simulink model "EDS1"  (R2023a)
settings: Solver=VariableStepAuto  StartTime=0.0  StopTime=600  RelTol=1e-3
undefined symbols (not defined in the file): Ion, Lithium
libraries: spsBatteryLib x2, spsDCMachineLib x2, spspowerguiLib x1
settings Model: PacingRate=0.011000  Creator=mluser  LastModifiedBy=Channaveera Gouda

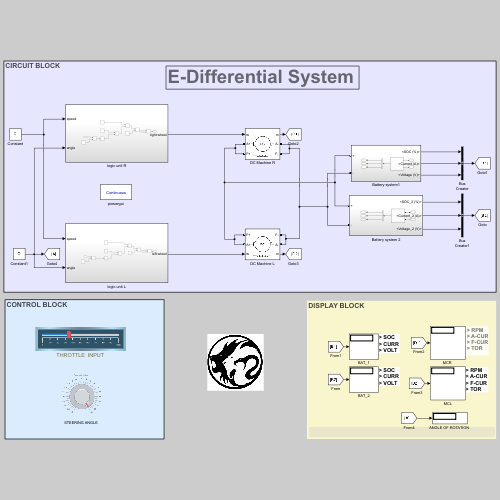
[thumbnail: Simulink's stored preview of the top-level diagram]
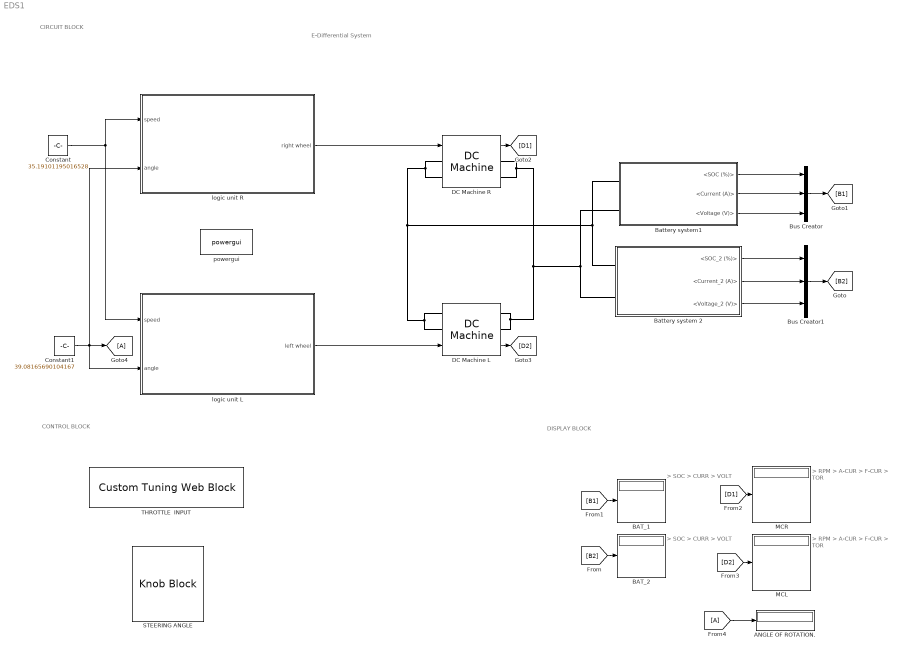
== system EDS1 ==
  note: CONTROL BLOCK
  note: DISPLAY BLOCK
  note: CIRCUIT BLOCK
  note: > RPM
      | > A-CUR
      | > F-CUR
      | > TOR
  note: > RPM
      | > A-CUR
      | > F-CUR
      | > TOR
  note: E-Differential System
  note: > SOC
      | > CURR
      | > VOLT
  note: > SOC
      | > CURR
      | > VOLT
  ANGLE OF ROTATION. : Display
  BAT_1 : Display
  BAT_2 : Display
  Battery system 2 : Subsystem
  Battery system1 : Subsystem
  Bus Creator : BusCreator  Inputs=3
  Bus Creator1 : BusCreator  Inputs=3
  Constant : Constant  Value=35.19101195016528
  Constant1 : Constant  Value=39.08165690104167
  DC Machine L : spsDCMachineLib/DC Machine  PresetModel=01: 5HP 240V 1750RPM Field:300V  MechanicalLoad=Speed w  FieldType=Wound  ShowDetailedParameters=on  MeasurementBus=off  RLa=[2.581 0.028]  RLf=[281.2 156]  Laf=0.9483  MachineConstant=Torque constant (N.m/A)  Ke=1.8  Kt=1.8  J=0.02215  Bm=0.002953  Tf=0.5161  w0=1  Ifinit=0  TsPowergui=0  TsBlock=-1
  DC Machine R : spsDCMachineLib/DC Machine  PresetModel=01: 5HP 240V 1750RPM Field:300V  MechanicalLoad=Speed w  FieldType=Wound  ShowDetailedParameters=on  MeasurementBus=off  RLa=[2.581 0.028]  RLf=[281.2 156]  Laf=0.9483  MachineConstant=Torque constant (N.m/A)  Ke=1.8  Kt=1.8  J=0.02215  Bm=0.002953  Tf=0.5161  w0=1  Ifinit=0  TsPowergui=0  TsBlock=-1
  From4 : From
  Goto4 : Goto
  MCL : Display
  "MCR " : Display
  STEERING ANGLE : KnobBlock  ScaleMin=-40  ScaleMax=40
  THROTTLE  INPUT : CustomTuningWebBlock  LabelPosition=Hide  ShowInitialText=on  Configuration="{\"components\":[{\"name\":\"LinearScaleComponent\",\"settings\":{\"bounds\":{\"max\":100,\"min\":0,\"tickInterval\":\"auto\"},\"internalTickHeightScaleFactor\":0.5,\"labelColor\":[255,255,200],\"labelFont\":{\"font\":\"Arial\",\"fontSize\":12},\"labelOffset\":0.05,\"labelTransparency\":1,\"needleImage\":{\"size\":[596,842],\"src\":\"data:image\\/svg+xml;base64,PD94bWwgdmVyc2lvbj0iMS4wIiBlbmNvZGluZz0idXRmLTgiPz4NCjwhLS0gR2VuZXJhdG9yOiBBZG9iZSBJbGx1c3RyYXRvciAyNS4wLjAsIFNWRyBFeHBvcnQgUGx1Zy1JbiAuIFNWRyBWZXJzaW9uOiA2LjAwIEJ1aWxkIDApICAtLT4NCjxzdmcgdmVyc2lvbj0iMS4xIg0KCSBpZD0ic3ZnOCIgeG1sbnM6Y2M9Imh0dHA6Ly9jcmVhdGl2ZWNvbW1vbnMub3JnL25zIyIgeG1sbnM6ZGM9Imh0dHA6Ly9wdXJsLm9yZy9kYy9lbGVtZW50cy8xLjEvIiB4bWxuczppbmtzY2FwZT0iaHR0cDovL3d3dy5pbmtzY2FwZS5vcmcvbmFtZXNw ...(+2420 chars)\",\"srcOrientation\":\"Right\"},\"needleOffset\":[-0.8044596912521441,-0.0642123287671233],\"needleSize\":{\"height\":0.4337797619047619,\"width\":0.07668067226890757},\"position\":[0.2829861111111111,0.04398634453781513,0.9196428571428571,0.6088789682539683],\"referencePoint\":\"auto\",\"scaleColors\":[],\"scaleColorsSize\":0.2,\"scaleDirection\":\"LR\",\"showLabels\":1,\"showMinorTicks\":0,\"showSpanLine\":1,\"showTicks\":1,\"tickColor\":[252,252,197],\"tickTransparency\":1,\"valueBarColor\":[0,114,189],\"valueBarOffset\":-0.27,\"valueBarSize\":0.1,\"valueBarTransparency\":1}},{\"name\":\"BackgroundImageComponent\",\"settings\":{\"image\":{\"size\":[380,101],\"src\":\"data:image\\/svg+xml;base64,PHN2ZyB4bWxucz0iaHR0cDovL3d3dy53My5vcmcvMjAwMC9zdmciIHhtbG5zOnhsaW5rPSJodHRwOi8vd3d3LnczLm9yZy8xOTk5L3hsaW5rIiB2aWV3Qm94PSIwIDAgMzgwIDEwMSI+PGRlZnM+PHN0eWxlPi5jbHMtMXtmaWxsOiMwMDJiNDI7fS5jbHMtMntmaWxsOiM0MjcwODI7fS5jbHMtM3tmaWxsOnVybCgjcmFkaWFsLWdyYWRpZW50KTt9LmNscy00e2ZpbGw6I2M4YzhjODtzdHJva2U6IzAwMDt9PC9zdHlsZT48cmFkaWFsR3JhZGllbnQgaWQ9InJhZGlhbC1ncmFkaWVudCIgY3g9IjE5MCIgY3k9IjUwLjUiIHI9IjI2OS4yMSIgZ3JhZGllbnRVbml0cz0idXNlclNwYWNlT25Vc2UiPjxzdG9wIG9mZnNldD0iMC4wMSIgc3RvcC1jb2xvcj0iIzNlNGY1OCIvPjxzdG9wIG9mZnNldD0iMC4wNiIgc3RvcC1jb2xvcj0iIzQ0NTc2MSIvPjxzdG9wIG9mZnNldD0iMC4xNSIgc3RvcC1jb2xvcj0iIzU1NmE3NiIvPjxzdG9wIG9mZnNldD0iMC4yNSIgc3RvcC1jb2xvcj0iIzZkODg5NSIvPjxzdG9wIG9mZnNldD0iMC4zOCIgc3RvcC1jb2xvcj0iIzhmYjJjMyIvPjxzdG9wIG9mZnNldD0iMC41MiIgc3RvcC1jb2xvcj0iI2I2ZTRmYSIvPjxzdG9wIG9mZnNldD0iMSIgc3RvcC1jb2xvcj0iIzE1NDY1NyIvPjwvcmFkaWFsR3JhZGllbnQ+PC9kZWZzPjxnIGlkPSJmcmFtZSI+PGcgaWQ9IkxheWVyXzIiIGRhdGEtbmFtZT0iTGF5ZXIgMiI+PGcgaWQ9IkxheWVyXzEtMiIgZGF0YS1uYW1lPSJMYXllciAxLTIiPjxyZWN0IGlkPSJyZWN0MTAzNiIgY2xhc3M9ImNscy0xIiB4PSIxMSIgeT0iMTEiIHdpZHRoPSIzNTgiIGhlaWdodD0iNzkiLz48cGF0aCBpZD0icGF0aDEwMzgiIGNsYXNzPSJjbHMtMiIgZD0iTTgsOFY5M0gzNzJWOFpNMzY5LDkwSDExVjExSDM2OVoiLz48cGF0aCBpZD0icGF0aDEwNDAiIGNsYXNzPSJjbHMtMyIgZD0iTTAsMFYxMDFIMzgwVjBaTTM3Miw5M0g4VjhIMzcyWiIvPjwvZz48L2c+PC9nPjxnIGlkPSJ0cmFjayI+PHBhdGggaWQ9InJlY3QxNjExIiBjbGFzcz0iY2xzLTQiIGQ9Ik0zMy4zNywyNi41OUgzNDYuNjNjNCwwLDcuMjUsMi42LDcuMjUsNS44MWgwYzAsMy4yMS0zLjI1LDUuODItNy4yNSw1LjgySDMzLjM3Yy00LDAtNy4yNS0yLjYxLTcuMjUtNS44MmgwQzI2LjEyLDI5LjE5LDI5LjM3LDI2LjU5LDMzLjM3LDI2LjU5WiIvPjwvZz48L3N2Zz4=\",\"srcOrientation\":\"horizontal\"},\"position\":[0,0,1,1],\"scaleMode\":\"0\"}},{\"name\":\"ForegroundImageComponent\",\"settings\":{\"image\":{\"size\":[0,0],\"src\":\"default\",\"srcOrientation\":[]},\"isForeground\":1,\"position\":[0,0,1,1],\"scaleMode\":\"0\"}}],\"settings\":{\"BindingType\":\"param\",\"aspectRatio\":3.7777777777777777,\"backgroundColor\":[0,0,0,\"1\"],\"backgroundOffset\":0,\"backgroundOpacity\":1,\"fixedAspectRatio\":\"on\",\"foregroundColor\":[252,252,196],\"orientation\":\"horizontal\",\"showBackgroundColor\":false,\"value\":0,\"version\":\"R2023a\"},\"type\":\"LinearGauge\"}"
  logic unit L : Subsystem
  logic unit R : Subsystem
  powergui : spspowerguiLib/powergui  Priority=1  SimulationMode=Continuous  SampleTime=50e-6  frequency=60  Iterations=50  frequencyindice=0  Pbase=100e6  ErrMax=1e-4  UnitsV=kV  UnitsW=MW  buscounter=0  FunctionMessages=off  echomessages=off  EnableUseOfTLC=off  CurrentSourceSwitches=off  DisableSnubberDevices=off  DisableRonSwitches=off  DisableVfSwitches=off  DisplayEquations=off  AutomaticDiscreteSolvers=off  SolverType=Tustin/Backward Euler (TBE)  Interpol=off  ExternalGateDelay=off  methode=off  Ts=100  x0status=blocks  SPID=on  SwTol=0  HookPort=off  NonlinearTolerance=1e-4  nMaxIteration=100  ContinueOnMaxIteration=off  RestoreLinks=warning  ResistiveCurrentMeasurement=off  Frange=[0:2:500]  Ylog=off  Xlog=on  ShowGrid=off  save=off  variable=ZData  structure=0  ZoomFFT=off  StartTime=0.0  cycles=1  DisplayStyle=1  fundamental=60  FreqAxis=off  MaxFrequency=1000  frequencyindicesteady=1  RmsSteady=1  display=off
  wires:
  Constant/1 -> logic unit L/1(speed), logic unit R/1(speed)
  Constant1/1 -> logic unit L/2(angle), Goto4/1, logic unit R/2(angle)
  logic unit L/1(left wheel) -> DC Machine L/1
  logic unit R/1(right wheel) -> DC Machine R/1
  Battery system1/3(<Voltage (V)>) -> Bus Creator/3
  Battery system1/2(<Current (A)>) -> Bus Creator/2
  Battery system1/1(<SOC (%)>) -> Bus Creator/1
  Battery system 2/2(<Current_2 (A)>) -> Bus Creator1/2
  Battery system 2/1(<SOC_2 (%)>) -> Bus Creator1/1
  Battery system 2/3(<Voltage_2 (V)>) -> Bus Creator1/3
  [B1] -> BAT_1/1
  Bus Creator/1 -> [B1]
  Bus Creator1/1 -> [B2]
  [B2] -> BAT_2/1
  DC Machine L/1 -> [D2]
  [D2] -> MCL/1
  DC Machine R/1 -> [D1]
  [D1] -> "MCR "/1
  From4/1 -> ANGLE OF ROTATION./1
  connections:
  DC Machine L/RConn2 -- DC Machine R/RConn2 -- DC Machine R/RConn1 -- Battery system 2/LConn2 -- Battery system1/LConn2 -- DC Machine L/RConn1
  DC Machine L/LConn2 -- DC Machine R/LConn2 -- DC Machine R/LConn1 -- Battery system 2/LConn1 -- Battery system1/LConn1 -- DC Machine L/LConn1

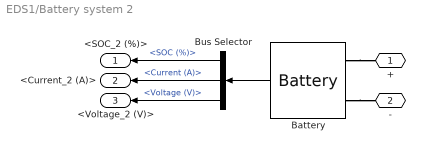
== system EDS1/Battery system 2 ==
  Battery : spsBatteryLib/Battery  BatType=Lithium-Ion  ShowTempParam=off  ThermalPreset=no  ShowAgeParam=off  NomV=75.6  NomQ=100  SOC=85  Batt_Tr=30  PresetModel=on  MaxQ=100  MinV=56.7  FullV=87.9974  Dis_rate=43.4783  R=0.00756  Normal_OP=90.4348  expZone="[81.6772      4.91304]"  current=[6.5 13 32.5]  Units=Time  Tci=20  NomT=20  T2=-30  MaxQ2=4.8  FullV2=7.1  Normal_OP2=5.655  expZone2="[6.58           1]"  Rca=0.6  ti=2000  Dp=0  Neq0=0  Tsim=1e6  Ta1=25  Qeol=5.4*0.9  Reol=0.013333*1.2  Char_age=[2.3478, 3]  Dis_age=[2.3478, 10]  N1=1500  N2=10500  N3=1000  N4=1400  Ta2=45  N5=950
  Bus Selector : BusSelector  OutputSignals=SOC (%),Current (A),Voltage (V)
  + : PMIOPort  Side=Left
  - : PMIOPort  Port=2  Side=Left
  <SOC_2 (%)> : Outport
  <Current_2 (A)> : Outport  Port=2
  <Voltage_2 (V)> : Outport  Port=3
  wires:
  Battery/1 -> Bus Selector/1
  Bus Selector/3 -> <Voltage_2 (V)>/1  "<Voltage (V)>"
  Bus Selector/2 -> <Current_2 (A)>/1  "<Current (A)>"
  Bus Selector/1 -> <SOC_2 (%)>/1  "<SOC (%)>"
  connections:
  Battery/LConn1 -- +/RConn1
  Battery/LConn2 -- -/RConn1

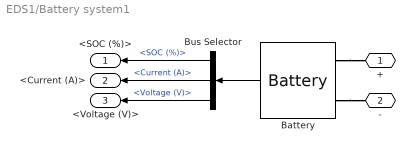
== system EDS1/Battery system1 ==
  Battery : spsBatteryLib/Battery  BatType=Lithium-Ion  ShowTempParam=off  ThermalPreset=no  ShowAgeParam=off  NomV=75.6  NomQ=100  SOC=85  Batt_Tr=30  PresetModel=on  MaxQ=100  MinV=56.7  FullV=87.9974  Dis_rate=43.4783  R=0.00756  Normal_OP=90.4348  expZone="[81.6772      4.91304]"  current=[6.5 13 32.5]  Units=Time  Tci=20  NomT=20  T2=-30  MaxQ2=4.8  FullV2=7.1  Normal_OP2=5.655  expZone2="[6.58           1]"  Rca=0.6  ti=2000  Dp=0  Neq0=0  Tsim=1e6  Ta1=25  Qeol=5.4*0.9  Reol=0.013333*1.2  Char_age=[2.3478, 3]  Dis_age=[2.3478, 10]  N1=1500  N2=10500  N3=1000  N4=1400  Ta2=45  N5=950
  Bus Selector : BusSelector  OutputSignals=SOC (%),Current (A),Voltage (V)
  + : PMIOPort  Side=Left
  - : PMIOPort  Port=2  Side=Left
  <SOC (%)> : Outport
  <Current (A)> : Outport  Port=2
  <Voltage (V)> : Outport  Port=3
  wires:
  Battery/1 -> Bus Selector/1
  Bus Selector/3 -> <Voltage (V)>/1  "<Voltage (V)>"
  Bus Selector/2 -> <Current (A)>/1  "<Current (A)>"
  Bus Selector/1 -> <SOC (%)>/1  "<SOC (%)>"
  connections:
  Battery/LConn1 -- +/RConn1
  Battery/LConn2 -- -/RConn1

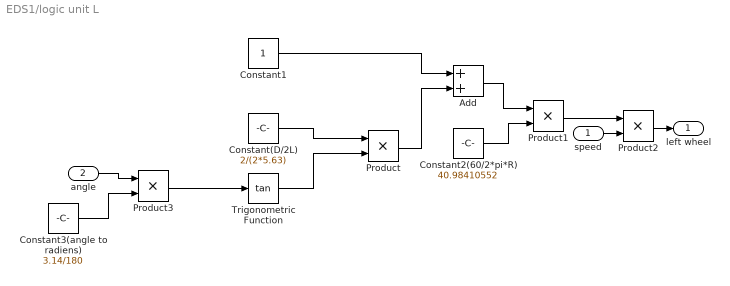
== system EDS1/logic unit L ==
  speed : Inport
  angle : Inport  Port=2
  Add : Sum
  Constant(D/2L) : Constant  Value=2/(2*5.63)
  Constant1 : Constant
  Constant2(60/2*pi*R) : Constant  Value=40.98410552
  Constant3(angle to radiens) : Constant  Value=3.14/180
  Product{,1..3} (4 alike) : Product
  Trigonometric Function : Trigonometry  Operator=tan
  left wheel : Outport
  wires:
  Product1/1 -> Product2/1
  Trigonometric Function/1 -> Product/2
  Product/1 -> Add/2
  Constant1/1 -> Add/1
  Constant(D/2L)/1 -> Product/1
  Constant2(60/2*pi*R)/1 -> Product1/2
  speed/1 -> Product2/2
  Add/1 -> Product1/1
  Product2/1 -> left wheel/1
  Constant3(angle to radiens)/1 -> Product3/2
  angle/1 -> Product3/1
  Product3/1 -> Trigonometric Function/1

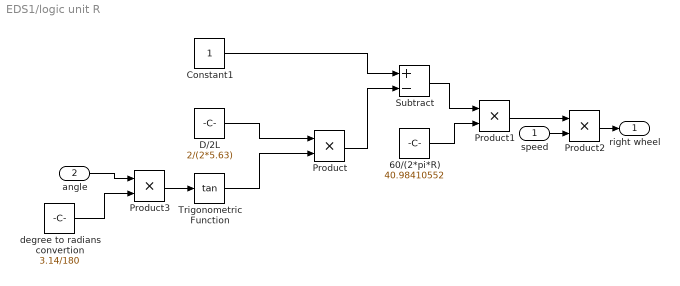
== system EDS1/logic unit R ==
  speed : Inport
  angle : Inport  Port=2
  60/(2*pi*R) : Constant  Value=40.98410552
  Constant1 : Constant
  D/2L : Constant  Value=2/(2*5.63)
  Product{,1..3} (4 alike) : Product
  Subtract : Sum  Inputs=+-
  Trigonometric Function : Trigonometry  Operator=tan
  degree to radians convertion : Constant  Value=3.14/180
  right wheel : Outport
  wires:
  Product1/1 -> Product2/1
  Trigonometric Function/1 -> Product/2
  Product/1 -> Subtract/2
  Constant1/1 -> Subtract/1
  D/2L/1 -> Product/1
  60/(2*pi*R)/1 -> Product1/2
  speed/1 -> Product2/2
  Subtract/1 -> Product1/1
  Product2/1 -> right wheel/1
  degree to radians convertion/1 -> Product3/2
  angle/1 -> Product3/1
  Product3/1 -> Trigonometric Function/1
